simulink model "lab_4_0x2810x29"  (R2024a)
settings: Solver=ode23t  StartTime=0.0  StopTime=2  RelTol=1e-3
undefined symbols (not defined in the file): magnitude
libraries: dspfdesign x3, commsynccomp2 x1
settings Model: Creator=CS Net Games  LastModifiedBy=hp
settings SolverCC: AlgebraicLoopSolver=TrustRegion
settings DebuggingCC: UnconnectedInputMsg=warning  UnconnectedOutputMsg=warning  UnconnectedLineMsg=warning
settings ModelReferenceCC: EnableRefExpFcnMdlSchedulingChecks=on
settings SFSimCC: CustomCodeUndefinedFunction=UseInterfaceOnly
settings RTWCC: GPUComputeCapability=3.5

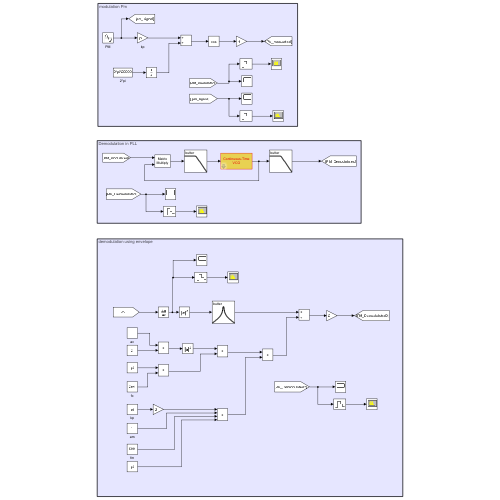
[thumbnail: Simulink's stored preview of the top-level diagram]
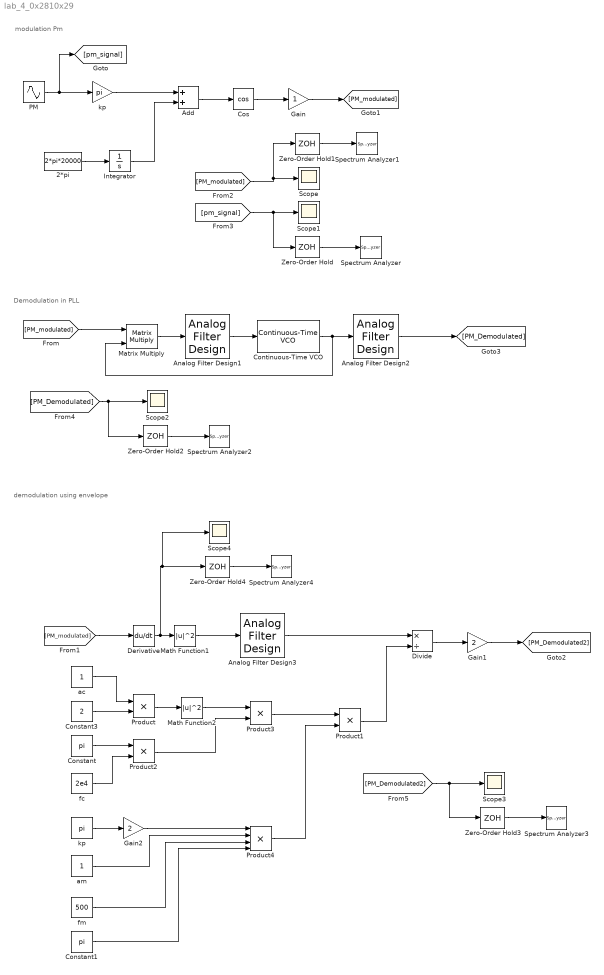
== system lab_4_0x2810x29 ==
  note: demodulation using envelope
  note: Demodulation in PLL
  note: modulation Pm
  "2*pi " : Constant  Value=2*pi*20000
  Add : Sum
  Analog Filter Design1 : dspfdesign/Analog Filter Design  method=Butterworth  filttype=Lowpass  N=8  Wlo=pi*2*600  Whi=80  Rp=2  Rs=40
  Analog Filter Design2 : dspfdesign/Analog Filter Design  method=Butterworth  filttype=Lowpass  N=8  Wlo=pi*2*600  Whi=80  Rp=2  Rs=40
  Analog Filter Design3 : dspfdesign/Analog Filter Design  method=Butterworth  filttype=Bandpass  N=8  Wlo=pi*2*475  Whi=pi*2*525  Rp=2  Rs=40
  Constant : Constant  Value=pi
  Constant1 : Constant  Value=pi
  Constant3 : Constant  Value=2
  Continuous-Time VCO : commsynccomp2/Continuous-Time VCO  Ac=1  Fc=500  Kc=1  Ph=0
  Cos : Trigonometry  Operator=cos
  Derivative : Derivative
  Divide : Product  Inputs=*/
  Gain : Gain
  Gain1 : Gain  Gain=2
  Gain2 : Gain  Gain=2
  Integrator : Integrator
  Math Function1 : Math  Operator=magnitude^2  SignedPower=on
  Math Function2 : Math  Operator=magnitude^2  SignedPower=on
  Matrix Multiply : Product  Multiplication=Matrix(*)
  "PM " : Sin  Frequency=500*pi*2  SampleTime=0
  Product{,1..3} (4 alike) : Product
  Product4 : Product  Inputs=4
  Scope{,1..4} (5 alike) : Scope
  Spectrum Analyzer : SpectrumAnalyzer  WindowPosition=[-128.000000,-14.000000,1282.000000,700.000000,]  ScopeFrameLocation=window  SpectrumType=RMS  Method=Welch  SampleRate=5000  Span=5000  StartFrequency=-2500  StopFrequency=2500  AveragingMethod=Running  SpectrumUnits=Vrms  Title=PM message signal  YLimits=[-0.0625,0.5625000000000009992]  AllowFFTLengthLessThanSamplesPerUpdate=on  DefaultConfigurationName=spbscopes.SpectrumAnalyzerBlockCfg  IsFrequencyInputMode=0  FrequencyVectorPort=0  FrequencyVectorFromPort=0  FrequencyInputRBWPort=0  FrequencyInputRBWFromPort=0
      settings: OpenAtSimulationStart=off
  Spectrum Analyzer1 : SpectrumAnalyzer  WindowPosition=[-128.000000,-14.000000,1282.000000,700.000000,]  ScopeFrameLocation=window  SpectrumType=RMS  Method=Welch  SampleRate=5000  Span=5000  StartFrequency=-2500  StopFrequency=2500  AveragingMethod=Running  SpectrumUnits=Vrms  Title=Modulated PM signal  YLimits=[-0.050210391821687246072,0.45189352639531149558]  AllowFFTLengthLessThanSamplesPerUpdate=on  DefaultConfigurationName=spbscopes.SpectrumAnalyzerBlockCfg  IsFrequencyInputMode=0  FrequencyVectorPort=0  FrequencyVectorFromPort=0  FrequencyInputRBWPort=0  FrequencyInputRBWFromPort=0
      settings: OpenAtSimulationStart=off
  Spectrum Analyzer2 : SpectrumAnalyzer  WindowPosition=[-128.000000,-14.000000,1282.000000,700.000000,]  ScopeFrameLocation=window  SpectrumType=RMS  Method=Welch  SampleRate=5000  AxesScaling=Manual  Span=5000  StartFrequency=-2500  StopFrequency=2500  AveragingMethod=Running  SpectrumUnits=Vrms  YLimits=[-0.060875356186415423287,0.54787821355457577699]  ShowLegend=on  ChannelNames="[\"PM demodulated by PLL\"]"  AllowFFTLengthLessThanSamplesPerUpdate=on  DefaultConfigurationName=spbscopes.SpectrumAnalyzerBlockCfg  IsFrequencyInputMode=0  FrequencyVectorPort=0  FrequencyVectorFromPort=0  FrequencyInputRBWPort=0  FrequencyInputRBWFromPort=0
      settings: OpenAtSimulationStart=off
  Spectrum Analyzer3 : SpectrumAnalyzer  WindowPosition=[-128.000000,-14.000000,1282.000000,700.000000,]  ScopeFrameLocation=window  SpectrumType=RMS  Method=Welch  SampleRate=5000  Span=5000  StartFrequency=-2500  StopFrequency=2500  AveragingMethod=Running  SpectrumUnits=Vrms  YLimits=[-0.056154252231000477413,0.50538827095485150398]  ShowLegend=on  ChannelNames="[\"PM modulated with envelope\"]"  AllowFFTLengthLessThanSamplesPerUpdate=on  DefaultConfigurationName=spbscopes.SpectrumAnalyzerBlockCfg  IsFrequencyInputMode=0  FrequencyVectorPort=0  FrequencyVectorFromPort=0  FrequencyInputRBWPort=0  FrequencyInputRBWFromPort=0
      settings: OpenAtSimulationStart=off
  Spectrum Analyzer4 : SpectrumAnalyzer  WindowPosition=[1.000000,1.000000,1280.000000,697.000000,]  ScopeFrameLocation=window  SpectrumType=RMS  Method=Welch  SampleRate=5000  Span=5000  StartFrequency=-2500  StopFrequency=2500  AveragingMethod=Running  SpectrumUnits=Vrms  YLimits=[-5004.4245299882031759,45064.563855548163701]  AllowFFTLengthLessThanSamplesPerUpdate=on  DefaultConfigurationName=spbscopes.SpectrumAnalyzerBlockCfg  IsFrequencyInputMode=0  FrequencyVectorPort=0  FrequencyVectorFromPort=0  FrequencyInputRBWPort=0  FrequencyInputRBWFromPort=0
      settings: OpenAtSimulationStart=off
  Zero-Order Hold : ZeroOrderHold  SampleTime=-1
  Zero-Order Hold1 : ZeroOrderHold  SampleTime=-1
  Zero-Order Hold2 : ZeroOrderHold  SampleTime=1/(10*5e2)
  Zero-Order Hold3 : ZeroOrderHold  SampleTime=1/(10*5e2)
  Zero-Order Hold4 : ZeroOrderHold  SampleTime=-1
  ac : Constant
  "am " : Constant
  fc : Constant  Value=2e4
  fm : Constant  Value=500
  kp : Gain  Gain=pi
  "kp " : Constant  Value=pi
  wires:
  Zero-Order Hold/1 -> Spectrum Analyzer/1
  [PM_modulated] -> Scope/1, Zero-Order Hold1/1
  Add/1 -> Cos/1
  Zero-Order Hold1/1 -> Spectrum Analyzer1/1
  Cos/1 -> Gain/1
  [pm_signal] -> Zero-Order Hold/1, Scope1/1
  Integrator/1 -> Add/2
  "2*pi "/1 -> Integrator/1
  Gain/1 -> [PM_modulated]
  kp/1 -> Add/1
  "PM "/1 -> [pm_signal], kp/1
  Matrix Multiply/1 -> Analog Filter Design1/1
  [PM_modulated] -> Matrix Multiply/1
  Analog Filter Design2/1 -> [PM_Demodulated]
  Analog Filter Design1/1 -> Continuous-Time VCO/1
  Zero-Order Hold2/1 -> Spectrum Analyzer2/1
  Continuous-Time VCO/1 -> Matrix Multiply/2, Analog Filter Design2/1
  [PM_Demodulated] -> Zero-Order Hold2/1, Scope2/1
  [PM_Demodulated2] -> Scope3/1, Zero-Order Hold3/1
  Gain2/1 -> Product4/1
  Zero-Order Hold3/1 -> Spectrum Analyzer3/1
  Gain1/1 -> [PM_Demodulated2]
  Divide/1 -> Gain1/1
  Product1/1 -> Divide/2
  "am "/1 -> Product4/2
  fm/1 -> Product4/3
  Constant/1 -> Product2/1
  Constant3/1 -> Product/2
  Product4/1 -> Product1/2
  Constant1/1 -> Product4/4
  "kp "/1 -> Gain2/1
  [PM_modulated] -> Derivative/1
  Math Function2/1 -> Product3/1
  Math Function1/1 -> Analog Filter Design3/1
  Product2/1 -> Product3/2
  Product3/1 -> Product1/1
  Analog Filter Design3/1 -> Divide/1
  ac/1 -> Product/1
  Product/1 -> Math Function2/1
  fc/1 -> Product2/2
  Derivative/1 -> Scope4/1, Zero-Order Hold4/1, Math Function1/1
  Zero-Order Hold4/1 -> Spectrum Analyzer4/1
